simulink library "lib_Convection_TurbIncompFlatPlateBL"  (R2015a)
settings: Solver=ode45  StartTime=0.0  StopTime=10.0  RelTol=1e-3
settings Model: Creator=jlkratz  LastModifiedBy=jlkratz

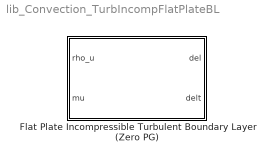
== system lib_Convection_TurbIncompFlatPlateBL ==
  Flat Plate Incompressible Turbulent Boundary Layer (Zero PG) : Subsystem  mask(TSAT: Flat Plate Incompressible Turbulent Boundary Layer (Zero PG)){x_M=1}
      mask prompts: x_M "x_M - Local position from the leading edge"
      mask help: This block approximates the boundary layer and thermal boundary layer thicknesses of incompressible turbulent flow over a flat plate with a pressure gradient of 0.
      mask Help: web(which('Convection_TSAT_TurbIncompFlatPlateBL.html'),'-helpbrowser')
      mask DialogControl Container3 Prompt: Parameters

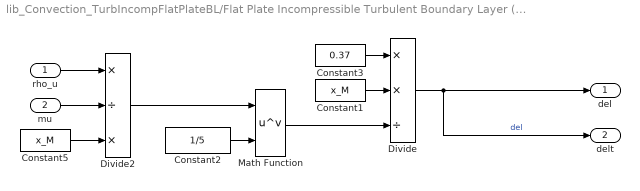
== system lib_Convection_TurbIncompFlatPlateBL/Flat Plate Incompressible Turbulent Boundary Layer (Zero PG) ==
  rho_u : Inport
  mu : Inport  Port=2
  Constant1 : Constant  Value=x_M
  Constant2 : Constant  Value=1/5
  Constant3 : Constant  Value=0.37
  Constant5 : Constant  Value=x_M
  Divide : Product  Inputs=**/
  Divide2 : Product  Inputs=*/*
  Math Function : Math  Operator=pow  SaturateOnIntegerOverflow=on
  del : Outport
  delt : Outport  Port=2
  wires:
  Divide/1 -> del/1, delt/1  "del"
  Math Function/1 -> Divide/3
  Constant2/1 -> Math Function/2
  Constant3/1 -> Divide/1
  Constant1/1 -> Divide/2
  rho_u/1 -> Divide2/1
  Constant5/1 -> Divide2/3
  mu/1 -> Divide2/2
  Divide2/1 -> Math Function/1
